simulink model "Suspension"  (R2020b)
settings: Solver=VariableStepAuto  StartTime=0.0  StopTime=100.0  RelTol=1e-3
undefined symbols (not defined in the file): b, k1, k2, m1, m2
settings Model: Creator=Shubham  LastModifiedBy=Shubham
settings DataIOCC: ExternalInput=[time, signal]  LoadExternalInput=on  SaveFormat=Array  ReturnWorkspaceOutputs=off  OutputSaveName=response

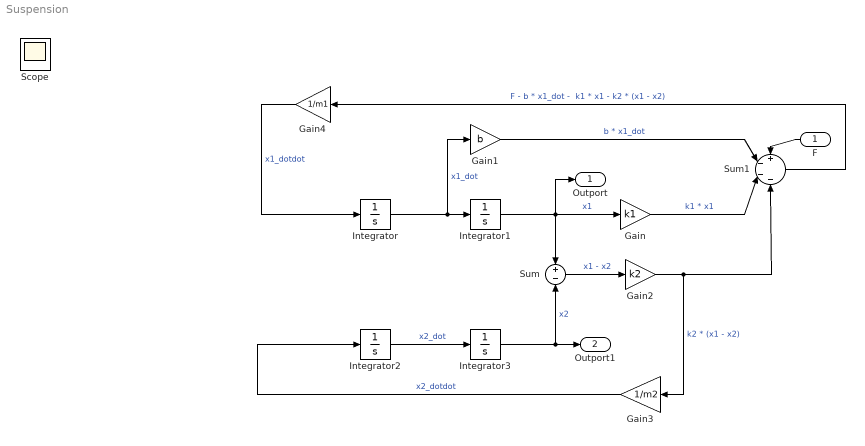
== system Suspension ==
  F : Inport
  Gain : Gain  Gain=k1
  Gain1 : Gain  Gain=b
  Gain2 : Gain  Gain=k2
  Gain3 : Gain  Gain=1/m2
  Gain4 : Gain  Gain=1/m1
  Integrator{,1..3} (4 alike) : Integrator
  Sum : Sum  Inputs=+-
  Sum1 : Sum  Inputs=+---
  Outport : Outport
  Outport1 : Outport  Port=2
  Scope : Scope
  wires:
  Integrator/1 -> Gain1/1, Integrator1/1  "x1_dot"
  Gain4/1 -> Integrator/1  "x1_dotdot"
  Integrator1/1 -> Outport/1, Sum/1, Gain/1  "x1"
  Integrator3/1 -> Outport1/1, Sum/2  "x2"
  Gain3/1 -> Integrator2/1  "x2_dotdot"
  Integrator2/1 -> Integrator3/1  "x2_dot"
  Gain/1 -> Sum1/3  "k1 * x1"
  Gain1/1 -> Sum1/2  "b * x1_dot"
  Sum/1 -> Gain2/1  "x1 - x2"
  Gain2/1 -> Sum1/4, Gain3/1  "k2 * (x1 - x2)"
  Sum1/1 -> Gain4/1  "F - b * x1_dot -  k1 * x1 - k2 * (x1 - x2)"
  F/1 -> Sum1/1
